simulink library "HY_General_Library"  (R2018b)
settings: Solver=ode45  StartTime=0.0  StopTime=10.0  RelTol=1e-3  EnableMultiTasking=on
undefined symbols (not defined in the file or in its folder): dT, Slope1, Slope2
libraries: simulink x63, $bdroot x4
(part 4 of 5)

== system HY_General_Library/PID_Blocks/IncrementalPID ==
  Err : Inport
  Kp : Inport  Port=2
  Ki : Inport  Port=3
  Kd : Inport  Port=4
  OutMax : Inport  Port=5
  OutMin : Inport  Port=6
  R : Inport  Port=7
  RV : Inport  Port=8
  Add : Sum  Inputs=+++
  Add1 : Sum  Inputs=+-
  Add2 : Sum
  Add3 : Sum  Inputs=+-
  Add4 : Sum  Inputs=+-
  Add5 : Sum
  Data Type Conversion : DataTypeConversion  OutDataTypeStr=single
  MinMax : MinMax  Inputs=2
  MinMax1 : MinMax  Function=max  Inputs=2
  Product : Product
  Product1 : Product
  Product2 : Product
  Switch : Switch  Criteria=u2 ~= 0
      settings: AttributesFormatString=%<Criteria>
  Unit Delay : UnitDelay  SampleTime=-1
      settings: AttributesFormatString=Init: %<X0>
  Unit Delay1 : UnitDelay  SampleTime=-1
      settings: AttributesFormatString=Init=%<X0>
  Unit Delay2 : UnitDelay  SampleTime=-1
      settings: AttributesFormatString=Init=%<X0>
  PIDOut : Outport
  POut : Outport  Port=2
  IOut : Outport  Port=3
  DOut : Outport  Port=4
  wires:
  Add2/1 -> Add1/1
  Kd/1 -> Product2/1
  Data Type Conversion/1 -> Unit Delay1/1, Add2/1, Product1/2, Add3/1
  Kp/1 -> Product/1
  Add4/1 -> Product2/2
  Ki/1 -> Product1/1
  Unit Delay1/1 -> Unit Delay2/1, Add1/2, Add4/2, Add3/2
  Add3/1 -> Product/2
  Product1/1 -> Add/2, IOut/1
  Product/1 -> Add/1, POut/1
  Product2/1 -> Add/3, DOut/1
  Err/1 -> Data Type Conversion/1
  OutMax/1 -> MinMax/1
  MinMax/1 -> MinMax1/1
  OutMin/1 -> MinMax1/2
  Unit Delay/1 -> Add5/2
  MinMax1/1 -> PIDOut/1, Unit Delay/1
  Add/1 -> Add5/1
  Add5/1 -> Switch/3
  Unit Delay2/1 -> Add2/2
  Add1/1 -> Add4/1
  Switch/1 -> MinMax/2
  R/1 -> Switch/2
  RV/1 -> Switch/1

== system HY_General_Library/PID_Blocks/PositionPID ==
  Err : Inport
  CtrlPropVal : Inport  Port=2
  CtrlIntgVal : Inport  Port=3
  CtrlDerivVal : Inport  Port=4
  UpperSatLimd : Inport  Port=5
  FfEnaFlag : Inport  Port=6
  FfVal : Inport  Port=7
  ThdMax : Inport  Port=8
  ThdMin : Inport  Port=9
  Reset : Inport  Port=10
  ResetVal : Inport  Port=11
  LowerSatLimd : Inport  Port=12
  Add : Sum  Inputs=+++
  Add3 : Sum  Inputs=+-
  Add4 : Sum
  MinMax : MinMax  Inputs=2
  MinMax1 : MinMax  Function=max  Inputs=2
  Product : Product
  Product2 : Product
  Subsystem1 : Subsystem
  Switch : Switch  Criteria=u2 ~= 0
  Unit Delay2 : UnitDelay  SampleTime=-1
  Output : Outport
  wires:
  Err/1 -> [Err], Product/1
  CtrlDerivVal/1 -> Product2/2
  [Err] -> Unit Delay2/1, Add3/1
  CtrlIntgVal/1 -> Subsystem1/5(CtrlIntgVal)
  ThdMax/1 -> MinMax/1
  Subsystem1/1(Out) -> Add/2
  Product/1 -> Add/1
  MinMax/1 -> MinMax1/1
  CtrlPropVal/1 -> Product/2
  FfVal/1 -> Add4/1
  Add/1 -> Switch/3, Add4/2
  Unit Delay2/1 -> Add3/2
  MinMax1/1 -> Output/1
  Add3/1 -> Product2/1
  Product2/1 -> Add/3
  ThdMin/1 -> MinMax1/2
  Reset/1 -> Subsystem1/1(Reset)
  [PreSat] -> Subsystem1/2(PreSat)
  UpperSatLimd/1 -> Subsystem1/3(UpperSatLimd)
  [Err] -> Subsystem1/4(Err)
  Switch/1 -> [PreSat], MinMax/2
  Add4/1 -> Switch/1
  FfEnaFlag/1 -> Switch/2
  ResetVal/1 -> Subsystem1/6(ResetVal)
  LowerSatLimd/1 -> Subsystem1/7(LowerSatLimd)

== system HY_General_Library/Time&Counter_Blocks/BounceTimer ==
  TmrEna : Inport
  Inc : Inport  Port=2
  MaxTime : Inport  Port=3
  Add : Sum
  Constant : Constant  Value=uint16(0)
  Multiport Switch1 : MultiPortSwitch  DataPortOrder=Zero-based contiguous  Inputs=2  zeroidx=on  OutDataTypeStr=double
  Relational Operator : RelationalOperator  OutDataTypeStr=boolean  RndMeth=Nearest
  Unit Delay1 : UnitDelay  SampleTime=-1
  TrigOut : Outport
  Timer : Outport  Port=2
  wires:
  Constant/1 -> Multiport Switch1/2
  TmrEna/1 -> Multiport Switch1/1
  MaxTime/1 -> Relational Operator/2
  Inc/1 -> Add/1
  Multiport Switch1/1 -> Add/2, Timer/1, Relational Operator/1
  Add/1 -> Unit Delay1/1
  Unit Delay1/1 -> Multiport Switch1/3
  Relational Operator/1 -> TrigOut/1

== system HY_General_Library/Time&Counter_Blocks/COUNTER ==
  E : Inport  OutDataTypeStr=boolean
  Constant1 : Constant  OutDataTypeStr=uint32
  Constant3 : Constant  Value=0  OutDataTypeStr=uint32
  Constant4 : Constant  Value=limit_value  OutDataTypeStr=uint32
  Min : MinMax  Inputs=2  SaturateOnIntegerOverflow=on
  Sum1 : Sum  SaturateOnIntegerOverflow=on
  Switch1 : Switch  Criteria=u2 ~= 0  Threshold=0.5  SaturateOnIntegerOverflow=on  InputSameDT=on
      settings: AttributesFormatString=%<Criteria>
  Unit Delay : UnitDelay  SampleTime=-1
      settings: AttributesFormatString=Init: %<X0>
  y : Outport
  wires:
  E/1 -> Switch1/2
  Sum1/1 -> Min/2
  Unit Delay/1 -> Sum1/1
  Constant3/1 -> Switch1/3
  Switch1/1 -> y/1, Unit Delay/1
  Min/1 -> Switch1/1
  Constant4/1 -> Min/1
  Constant1/1 -> Sum1/2

== system HY_General_Library/Time&Counter_Blocks/COUNTER_H ==
  E : Inport  OutDataTypeStr=boolean
  R : Inport  Port=2  OutDataTypeStr=boolean
  Constant1 : Constant  OutDataTypeStr=uint32
  Constant2 : Constant  Value=0  OutDataTypeStr=uint32
  Constant3 : Constant  Value=0  OutDataTypeStr=uint32
  Constant4 : Constant  Value=limit_value  OutDataTypeStr=uint32
  MinMax : MinMax  Inputs=2  SaturateOnIntegerOverflow=on
  Sum1 : Sum  SaturateOnIntegerOverflow=on
  Switch : Switch  Criteria=u2 ~= 0  Threshold=0.5
  Switch1 : Switch  Criteria=u2 ~= 0  Threshold=0.5  SaturateOnIntegerOverflow=on  InputSameDT=on
      settings: AttributesFormatString=%<Criteria>
  Unit Delay : UnitDelay  SampleTime=-1
      settings: AttributesFormatString=Init: %<X0>
  y : Outport
  wires:
  Unit Delay/1 -> Sum1/2
  Switch/1 -> Sum1/1
  Constant3/1 -> Switch1/1
  MinMax/1 -> Switch1/3
  Constant4/1 -> MinMax/1
  Switch1/1 -> Unit Delay/1, y/1
  Constant2/1 -> Switch/3
  Sum1/1 -> MinMax/2
  Constant1/1 -> Switch/1
  E/1 -> Switch/2
  R/1 -> Switch1/2

== system HY_General_Library/Time&Counter_Blocks/STOPWATCH_RE ==
  E : Inport  OutDataTypeStr=boolean
  R : Inport  Port=2  OutDataTypeStr=boolean
  dT : Inport  Port=3
  Constant1 : Constant  Value=0.0  OutDataTypeStr=Inherit: Inherit via back propagation
  Sum1 : Sum  SaturateOnIntegerOverflow=on
  Switch : Switch  Criteria=u2 ~= 0  SaturateOnIntegerOverflow=on  InputSameDT=on
  Switch1 : Switch  Criteria=u2 ~= 0  SaturateOnIntegerOverflow=on  InputSameDT=on
  Unit Delay1 : UnitDelay  SampleTime=-1
      settings: AttributesFormatString=<initial=%<x0>>
  t : Outport
  wires:
  Sum1/1 -> Switch1/1
  Unit Delay1/1 -> Switch1/3, Sum1/2
  R/1 -> Switch/2
  Constant1/1 -> Switch/1
  E/1 -> Switch1/2
  Switch1/1 -> Switch/3
  Switch/1 -> t/1, Unit Delay1/1
  dT/1 -> Sum1/1

== system HY_General_Library/Time&Counter_Blocks/TIMER ==
  T : Inport
  S : Inport  Port=2  OutDataTypeStr=boolean
  dT : Inport  Port=3
  Constant3 : Constant  Value=0.0001  OutDataTypeStr=Inherit: Inherit via back propagation
  Constant5 : Constant  Value=0  OutDataTypeStr=Inherit: Inherit via back propagation
  Logical Operator1 : Logic  Operator=NOT  Inputs=1  OutDataTypeStr=boolean
  Logical Operator2 : Logic  OutDataTypeStr=boolean
  Logical Operator4 : Logic  Operator=NOT  Inputs=1  OutDataTypeStr=boolean
  Logical Operator5 : Logic  OutDataTypeStr=boolean
  Logical Operator7 : Logic  Operator=OR  OutDataTypeStr=boolean
  MinMax : MinMax  Inputs=2  SaturateOnIntegerOverflow=on  InputSameDT=on
  Relational Operator : RelationalOperator  Operator=<=  OutDataTypeStr=boolean  RndMeth=Nearest  InputSameDT=on
  Sum : Sum  SaturateOnIntegerOverflow=on
  Sum1 : Sum  SaturateOnIntegerOverflow=on
  Switch2 : Switch  Criteria=u2 ~= 0  Threshold=0.5  SaturateOnIntegerOverflow=on  InputSameDT=on
  Switch3 : Switch  Criteria=u2 ~= 0  Threshold=0.5  SaturateOnIntegerOverflow=on  InputSameDT=on
  Unit Delay : UnitDelay  SampleTime=-1
      settings: AttributesFormatString=<initial=%<x0>>
  Unit Delay1 : UnitDelay  SampleTime=-1
      settings: AttributesFormatString=<initial=%<x0>>
  Unit Delay2 : UnitDelay  SampleTime=-1
      settings: AttributesFormatString=<initial=%<x0>>
  y : Outport
  t : Outport  Port=2
  wires:
  Logical Operator1/1 -> Logical Operator7/2
  Logical Operator4/1 -> Logical Operator5/2
  T/1 -> Switch3/1
  Sum/1 -> Switch2/3
  Unit Delay1/1 -> Logical Operator4/1
  Constant5/1 -> Switch2/1
  Sum1/1 -> Relational Operator/2
  Logical Operator2/1 -> y/1
  Constant3/1 -> Sum1/1
  Relational Operator/1 -> Logical Operator2/2
  S/1 -> Logical Operator2/1, Unit Delay1/1, Logical Operator5/1, Logical Operator1/1
  Switch3/1 -> Relational Operator/1, MinMax/1, Unit Delay2/1  "sampled_target_time"
  Unit Delay2/1 -> Switch3/3
  Switch2/1 -> MinMax/2
  Logical Operator7/1 -> Switch2/2
  dT/1 -> Sum/1
  Logical Operator5/1 -> Switch3/2, Logical Operator7/1  "edge"
  Unit Delay/1 -> Sum/2  "timer_value_old"
  MinMax/1 -> t/1, Unit Delay/1, Sum1/2

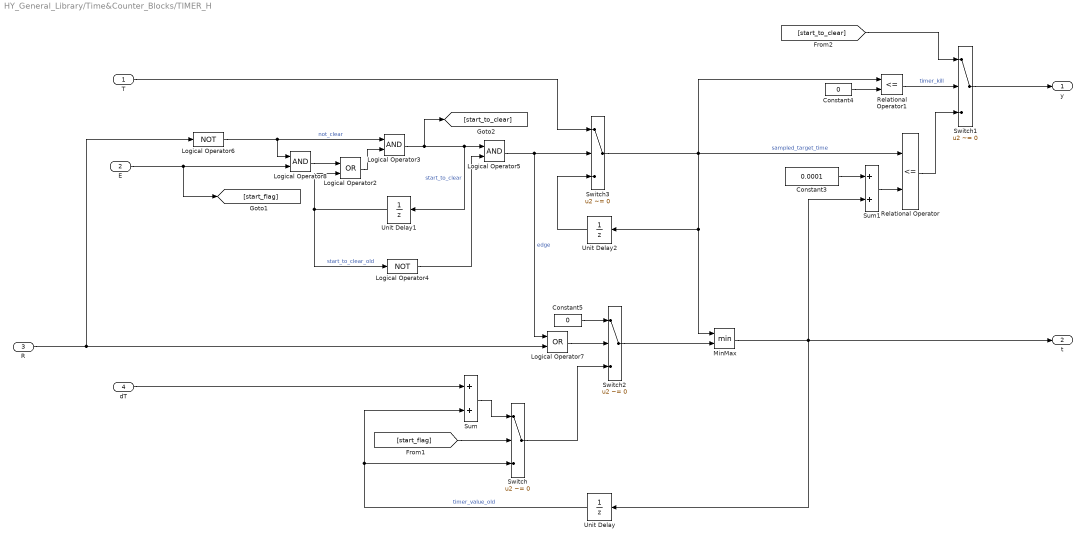
== system HY_General_Library/Time&Counter_Blocks/TIMER_H ==
  T : Inport
  E : Inport  Port=2  OutDataTypeStr=boolean
  R : Inport  Port=3  OutDataTypeStr=boolean
  dT : Inport  Port=4
  Constant3 : Constant  Value=0.0001  OutDataTypeStr=Inherit: Inherit via back propagation
  Constant4 : Constant  Value=0  OutDataTypeStr=Inherit: Inherit via back propagation
  Constant5 : Constant  Value=0  OutDataTypeStr=Inherit: Inherit via back propagation
  Logical Operator2 : Logic  Operator=OR  OutDataTypeStr=boolean
  Logical Operator3 : Logic  OutDataTypeStr=boolean
  Logical Operator4 : Logic  Operator=NOT  Inputs=1  OutDataTypeStr=boolean
  Logical Operator5 : Logic  OutDataTypeStr=boolean
  Logical Operator6 : Logic  Operator=NOT  Inputs=1  OutDataTypeStr=boolean
  Logical Operator7 : Logic  Operator=OR  OutDataTypeStr=boolean
  Logical Operator8 : Logic  OutDataTypeStr=boolean
  MinMax : MinMax  Inputs=2  SaturateOnIntegerOverflow=on  InputSameDT=on
  Relational Operator : RelationalOperator  Operator=<=  OutDataTypeStr=boolean  RndMeth=Nearest  InputSameDT=on
  Relational Operator1 : RelationalOperator  Operator=<=  OutDataTypeStr=boolean  RndMeth=Nearest  InputSameDT=on
  Sum : Sum  SaturateOnIntegerOverflow=on
  Sum1 : Sum  SaturateOnIntegerOverflow=on
  Switch{,1..3} (4 alike) : Switch  Criteria=u2 ~= 0  Threshold=0.5  SaturateOnIntegerOverflow=on  InputSameDT=on
  Unit Delay : UnitDelay  SampleTime=-1
      settings: AttributesFormatString=<initial=%<x0>>
  Unit Delay1 : UnitDelay  SampleTime=-1
      settings: AttributesFormatString=<initial=%<x0>>
  Unit Delay2 : UnitDelay  SampleTime=-1
      settings: AttributesFormatString=<initial=%<x0>>
  y : Outport
  t : Outport  Port=2
  wires:
  [start_to_clear] -> Switch1/1
  E/1 -> Logical Operator8/2, [start_flag]
  MinMax/1 -> Sum1/2, Unit Delay/1, t/1
  Unit Delay/1 -> Switch/3, Sum/2  "timer_value_old"
  R/1 -> Logical Operator6/1, Logical Operator7/2
  Logical Operator8/1 -> Logical Operator2/1
  [start_flag] -> Switch/2
  Logical Operator6/1 -> Logical Operator8/1, Logical Operator3/1  "not_clear"
  T/1 -> Switch3/1
  Logical Operator5/1 -> Logical Operator7/1, Switch3/2  "edge"
  Logical Operator4/1 -> Logical Operator5/2
  Unit Delay1/1 -> Logical Operator4/1, Logical Operator2/2  "start_to_clear_old"
  Logical Operator3/1 -> [start_to_clear], Logical Operator5/1, Unit Delay1/1  "start_to_clear"
  Logical Operator2/1 -> Logical Operator3/2
  dT/1 -> Sum/1
  Sum/1 -> Switch/1
  Switch/1 -> Switch2/3
  Logical Operator7/1 -> Switch2/2
  Switch2/1 -> MinMax/2
  Unit Delay2/1 -> Switch3/3
  Switch3/1 -> Relational Operator1/1, Unit Delay2/1, MinMax/1, Relational Operator/1  "sampled_target_time"
  Relational Operator/1 -> Switch1/3
  Constant3/1 -> Sum1/1
  Relational Operator1/1 -> Switch1/2  "timer_kill"
  Switch1/1 -> y/1
  Constant4/1 -> Relational Operator1/2
  Sum1/1 -> Relational Operator/2
  Constant5/1 -> Switch2/1

== system HY_General_Library/Time&Counter_Blocks/TIME_Y ==
  T : Inport
  S : Inport  Port=2  OutDataTypeStr=boolean
  dT : Inport  Port=3
  Constant3 : Constant  Value=0.0001  OutDataTypeStr=Inherit: Inherit via back propagation
  Constant5 : Constant  Value=0  OutDataTypeStr=Inherit: Inherit via back propagation
  Logical Operator1 : Logic  Operator=NOT  Inputs=1  OutDataTypeStr=boolean
  Logical Operator2 : Logic  OutDataTypeStr=boolean
  Logical Operator4 : Logic  Operator=NOT  Inputs=1  OutDataTypeStr=boolean
  Logical Operator5 : Logic  OutDataTypeStr=boolean
  Logical Operator7 : Logic  Operator=OR  OutDataTypeStr=boolean
  MinMax : MinMax  Inputs=2  SaturateOnIntegerOverflow=on  InputSameDT=on
  Relational Operator : RelationalOperator  Operator=<=  OutDataTypeStr=boolean  RndMeth=Nearest  InputSameDT=on
  Sum : Sum  SaturateOnIntegerOverflow=on
  Sum1 : Sum  SaturateOnIntegerOverflow=on
  Switch2 : Switch  Criteria=u2 ~= 0  Threshold=0.5  SaturateOnIntegerOverflow=on  InputSameDT=on
  Switch3 : Switch  Criteria=u2 ~= 0  Threshold=0.5  SaturateOnIntegerOverflow=on  InputSameDT=on
  Unit Delay : UnitDelay  SampleTime=-1
      settings: AttributesFormatString=<initial=%<x0>>
  Unit Delay1 : UnitDelay  SampleTime=-1
      settings: AttributesFormatString=<initial=%<x0>>
  Unit Delay2 : UnitDelay  SampleTime=-1
      settings: AttributesFormatString=<initial=%<x0>>
  y : Outport
  wires:
  MinMax/1 -> Sum1/2, Unit Delay/1
  Unit Delay/1 -> Sum/2  "timer_value_old"
  Logical Operator5/1 -> Logical Operator7/1, Switch3/2  "edge"
  dT/1 -> Sum/1
  Logical Operator7/1 -> Switch2/2
  Switch2/1 -> MinMax/2
  Unit Delay2/1 -> Switch3/3
  Switch3/1 -> Unit Delay2/1, MinMax/1, Relational Operator/1  "sampled_target_time"
  S/1 -> Logical Operator1/1, Logical Operator5/1, Unit Delay1/1, Logical Operator2/1
  Relational Operator/1 -> Logical Operator2/2
  Constant3/1 -> Sum1/1
  Logical Operator2/1 -> y/1
  Sum1/1 -> Relational Operator/2
  Constant5/1 -> Switch2/1
  Unit Delay1/1 -> Logical Operator4/1
  Sum/1 -> Switch2/3
  T/1 -> Switch3/1
  Logical Operator4/1 -> Logical Operator5/2
  Logical Operator1/1 -> Logical Operator7/2

== system HY_General_Library/Time&Counter_Blocks/TurnOffDelay ==
  u : Inport
  T : Inport  Port=2
  dT : Inport  Port=3
  Dif : Sum  Inputs=+-  SaturateOnIntegerOverflow=on
  Logical Operator1 : Logic  Operator=OR  OutDataTypeStr=boolean
  Relational Operator : RelationalOperator  Operator=>  OutDataTypeStr=boolean  RndMeth=Nearest  InputSameDT=on
  Switch : Switch  Criteria=u2 ~= 0  SaturateOnIntegerOverflow=on  InputSameDT=on
  Switch1 : Switch  Criteria=u2 ~= 0  SaturateOnIntegerOverflow=on  InputSameDT=on
  Unit Delay1 : UnitDelay  SampleTime=-1
      settings: AttributesFormatString=<initial=%<x0>>
  Zero_C : Constant  Value=0.0  OutDataTypeStr=Inherit: Inherit via back propagation
  y : Outport  InitialOutput=0
  wires:
  u/1 -> Switch/2, Logical Operator1/2
  Unit Delay1/1 -> Dif/1, Relational Operator/1, Switch1/3
  T/1 -> Switch/1
  Relational Operator/1 -> Logical Operator1/1, Switch1/2
  Logical Operator1/1 -> y/1
  Switch/1 -> Unit Delay1/1
  Zero_C/1 -> Relational Operator/2
  Switch1/1 -> Switch/3
  dT/1 -> Dif/2
  Dif/1 -> Switch1/1

== system HY_General_Library/Time&Counter_Blocks/TurnOffDelayCnt ==
  u : Inport
  Cnt : Inport  Port=2
  Constant1 : Constant  Value=0  OutDataTypeStr=Inherit: Inherit via back propagation
  Constant2 : Constant  OutDataTypeStr=Inherit: Inherit via back propagation
  Constant3 : Constant  Value=0  OutDataTypeStr=Inherit: Inherit via back propagation
  Data Type Duplicate : DataTypeDuplicate  NumInputPorts=4
  Logical Operator : Logic  OutDataTypeStr=boolean
  Logical Operator1 : Logic  OutDataTypeStr=boolean
  Logical Operator2 : Logic  Operator=NOT  OutDataTypeStr=boolean
  RelationalOperator : RelationalOperator  RndMeth=Nearest  InputSameDT=on
  Sum : Sum  SaturateOnIntegerOverflow=on
  Switch1 : Switch  Criteria=u2 ~= 0  SaturateOnIntegerOverflow=on  InputSameDT=on
      settings: AttributesFormatString=%<Criteria>
  Switch4 : Switch  Criteria=u2 ~= 0  SaturateOnIntegerOverflow=on  InputSameDT=on
      settings: AttributesFormatString=%<Criteria>
  Unit Delay : UnitDelay  SampleTime=-1
      settings: AttributesFormatString=Init: %<X0>
  Unit Delay1 : UnitDelay  SampleTime=-1
      settings: AttributesFormatString=Init: %<X0>
  y : Outport
  wires:
  [u] -> Logical Operator/2
  Switch1/1 -> Sum/1
  Constant3/1 -> Switch1/3, Data Type Duplicate/2
  [u] -> Switch1/2
  Unit Delay/1 -> Switch1/1
  Switch4/1 -> Sum/2
  Constant2/1 -> Switch4/1, Data Type Duplicate/3
  Constant1/1 -> Switch4/3, Data Type Duplicate/4
  Logical Operator2/1 -> Logical Operator1/1
  Logical Operator1/1 -> Switch4/2
  Unit Delay1/1 -> Logical Operator2/1
  Cnt/1 -> RelationalOperator/2, Data Type Duplicate/1
  Sum/1 -> Unit Delay/1, RelationalOperator/1
  Logical Operator/1 -> y/1
  RelationalOperator/1 -> Logical Operator/1, Unit Delay1/1
  u/1 -> [u], Logical Operator1/2

== system HY_General_Library/Time&Counter_Blocks/TurnOffDelay_R ==
  u : Inport
  R : Inport  Port=2
  T : Inport  Port=3
  dT : Inport  Port=4
  Data Type Duplicate : DataTypeDuplicate  NumInputPorts=4
  Dif : Sum  Inputs=+-  SaturateOnIntegerOverflow=on
  Logical Operator1 : Logic  Operator=OR  OutDataTypeStr=boolean
  Logical Operator2 : Logic
  Logical Operator3 : Logic  Operator=NOT  Inputs=1  AllPortsSameDT=off  OutDataTypeStr=boolean
  Relational Operator : RelationalOperator  Operator=>  OutDataTypeStr=boolean  RndMeth=Nearest  InputSameDT=on
  Switch : Switch  Criteria=u2 ~= 0  SaturateOnIntegerOverflow=on  InputSameDT=on
      settings: AttributesFormatString=%<Criteria>
  Switch1 : Switch  Criteria=u2 ~= 0  SaturateOnIntegerOverflow=on  InputSameDT=on
      settings: AttributesFormatString=%<Criteria>
  Switch2 : Switch  Criteria=u2 ~= 0  SaturateOnIntegerOverflow=on  InputSameDT=on
      settings: AttributesFormatString=%<Criteria>
  Unit Delay1 : UnitDelay  SampleTime=-1
      settings: AttributesFormatString=Init: %<X0>
  Zero_C : Constant  Value=0  OutDataTypeStr=Inherit: Inherit via back propagation
  Zero_C1 : Constant  Value=0  OutDataTypeStr=single
      settings: AttributesFormatString=%<OutDataTypeStr>
  y : Outport  InitialOutput=0
  wires:
  Logical Operator2/1 -> Logical Operator1/2, Switch/2
  Switch2/1 -> Switch1/3, Relational Operator/1, Dif/1
  T/1 -> Switch/1, Data Type Duplicate/4
  Relational Operator/1 -> Logical Operator1/1, Switch1/2
  Logical Operator1/1 -> y/1
  Switch/1 -> Unit Delay1/1
  Zero_C/1 -> Data Type Duplicate/1, Relational Operator/2
  Switch1/1 -> Switch/3
  dT/1 -> Data Type Duplicate/2, Dif/2
  Dif/1 -> Switch1/1
  u/1 -> Logical Operator2/2
  Logical Operator3/1 -> Logical Operator2/1
  R/1 -> Logical Operator3/1, Switch2/2
  Unit Delay1/1 -> Switch2/3
  Zero_C1/1 -> Switch2/1, Data Type Duplicate/3

== system HY_General_Library/Time&Counter_Blocks/TurnOnDelay ==
  u : Inport
  T : Inport  Port=2
  dT : Inport  Port=3
  Constant1 : Constant  Value=0.0  OutDataTypeStr=Inherit: Inherit via back propagation
  Logical Operator : Logic  OutDataTypeStr=boolean
  Logical Operator2 : Logic  Operator=NOT  Inputs=1  AllPortsSameDT=off  OutDataTypeStr=boolean
  Logical Operator3 : Logic  Operator=NOT  Inputs=1  AllPortsSameDT=off  OutDataTypeStr=boolean
  Logical Operator4 : Logic  Operator=NOT  Inputs=1  AllPortsSameDT=off  OutDataTypeStr=boolean
  Relational Operator2 : RelationalOperator  Operator=>  OutDataTypeStr=boolean  RndMeth=Nearest  InputSameDT=on
  Sum : Sum  Inputs=+-  SaturateOnIntegerOverflow=on
  Switch : Switch  Criteria=u2 ~= 0  SaturateOnIntegerOverflow=on  InputSameDT=on
      settings: AttributesFormatString=%<Criteria>
  Switch4 : Switch  Criteria=u2 ~= 0  SaturateOnIntegerOverflow=on  InputSameDT=on
      settings: AttributesFormatString=%<Criteria>
  Unit Delay : UnitDelay  SampleTime=-1
      settings: AttributesFormatString=Init: %<X0>
  y : Outport
  wires:
  Logical Operator2/1 -> Switch/2
  Switch4/1 -> Unit Delay/1
  Sum/1 -> Switch/3
  dT/1 -> Sum/2
  Constant1/1 -> Relational Operator2/2
  Relational Operator2/1 -> Logical Operator2/1, Logical Operator3/1
  u/1 -> Logical Operator4/1, Logical Operator/2
  Logical Operator/1 -> y/1
  Switch/1 -> Switch4/3
  Logical Operator3/1 -> Logical Operator/1
  Logical Operator4/1 -> Switch4/2
  T/1 -> Switch4/1
  Unit Delay/1 -> Relational Operator2/1, Switch/1, Sum/1

== system HY_General_Library/Time&Counter_Blocks/TurnOnDelayCnt ==
  u : Inport
  Cnt : Inport  Port=2
  Constant1 : Constant  Value=0  OutDataTypeStr=Inherit: Inherit via back propagation
  Constant2 : Constant  OutDataTypeStr=Inherit: Inherit via back propagation
  Constant3 : Constant  Value=0  OutDataTypeStr=Inherit: Inherit via back propagation
  Data Type Duplicate : DataTypeDuplicate  NumInputPorts=4
  Logical Operator : Logic  OutDataTypeStr=boolean
  Logical Operator1 : Logic  OutDataTypeStr=boolean
  Logical Operator2 : Logic  Operator=NOT  OutDataTypeStr=boolean
  RelationalOperator : RelationalOperator  RndMeth=Nearest  InputSameDT=on
  Sum : Sum  SaturateOnIntegerOverflow=on
  Switch1 : Switch  Criteria=u2 ~= 0  SaturateOnIntegerOverflow=on  InputSameDT=on
      settings: AttributesFormatString=%<Criteria>
  Switch4 : Switch  Criteria=u2 ~= 0  SaturateOnIntegerOverflow=on  InputSameDT=on
      settings: AttributesFormatString=%<Criteria>
  Unit Delay : UnitDelay  SampleTime=-1
      settings: AttributesFormatString=Init: %<X0>
  Unit Delay1 : UnitDelay  SampleTime=-1
      settings: AttributesFormatString=Init: %<X0>
  y : Outport
  wires:
  u/1 -> Logical Operator1/2, [u]
  RelationalOperator/1 -> Unit Delay1/1, Logical Operator/1
  Logical Operator/1 -> y/1
  Sum/1 -> RelationalOperator/1, Unit Delay/1
  Cnt/1 -> Data Type Duplicate/1, RelationalOperator/2
  Unit Delay1/1 -> Logical Operator2/1
  Logical Operator1/1 -> Switch4/2
  Logical Operator2/1 -> Logical Operator1/1
  Constant1/1 -> Data Type Duplicate/4, Switch4/3
  Constant2/1 -> Data Type Duplicate/3, Switch4/1
  Switch4/1 -> Sum/2
  Unit Delay/1 -> Switch1/1
  [u] -> Switch1/2
  Constant3/1 -> Data Type Duplicate/2, Switch1/3
  Switch1/1 -> Sum/1
  [u] -> Logical Operator/2

== system HY_General_Library/Time&Counter_Blocks/TurnOnDelay_IV ==
  u : Inport
  T : Inport  Port=2
  dT : Inport  Port=3
  IV : Inport  Port=4
  Constant : Constant  Value=boolean(0)  OutDataTypeStr=boolean
  Constant1 : Constant  Value=0.0  OutDataTypeStr=Inherit: Inherit via back propagation
  Logical Operator : Logic  OutDataTypeStr=boolean
  Logical Operator2 : Logic  Operator=NOT  Inputs=1  AllPortsSameDT=off  OutDataTypeStr=boolean
  Logical Operator3 : Logic  Operator=NOT  Inputs=1  AllPortsSameDT=off  OutDataTypeStr=boolean
  Logical Operator4 : Logic  Operator=NOT  Inputs=1  AllPortsSameDT=off  OutDataTypeStr=boolean
  Relational Operator2 : RelationalOperator  Operator=>  RndMeth=Nearest  InputSameDT=on
  Sum : Sum  Inputs=+-  SaturateOnIntegerOverflow=on
  Switch : Switch  Criteria=u2 ~= 0  SaturateOnIntegerOverflow=on  InputSameDT=on
  Switch1 : Switch  Criteria=u2 ~= 0  SaturateOnIntegerOverflow=on  InputSameDT=on
  Switch4 : Switch  Criteria=u2 ~= 0  SaturateOnIntegerOverflow=on  InputSameDT=on
  Unit Delay : UnitDelay  SampleTime=-1
      settings: AttributesFormatString=<initial=%<x0>>
  Unit Delay1 : UnitDelay  InitialCondition=1  SampleTime=-1
  y : Outport
  wires:
  Unit Delay/1 -> Sum/1, Switch/1, Relational Operator2/1
  T/1 -> Switch4/1
  Logical Operator4/1 -> Switch4/2
  Logical Operator3/1 -> Logical Operator/1
  Switch/1 -> Switch4/3
  Switch1/1 -> y/1
  u/1 -> Logical Operator/2, Logical Operator4/1
  Relational Operator2/1 -> Logical Operator3/1, Logical Operator2/1
  Constant1/1 -> Relational Operator2/2
  dT/1 -> Sum/2
  Sum/1 -> Switch/3
  Switch4/1 -> Unit Delay/1
  Logical Operator2/1 -> Switch/2
  Logical Operator/1 -> Switch1/3
  Unit Delay1/1 -> Switch1/2
  Constant/1 -> Unit Delay1/1
  IV/1 -> Switch1/1

== system HY_General_Library/Trigger_Blocks/EVENT ==
  Constant1 : Constant  Value=EventTime  OutDataTypeStr=Inherit: Inherit via back propagation
  Constant2 : Constant  Value=0  OutDataTypeStr=Inherit: Inherit via back propagation
  Constant3 : Constant  Value=0.0001  OutDataTypeStr=Inherit: Inherit via back propagation
  Constant4 : Constant  Value=SampleTime  OutDataTypeStr=Inherit: Inherit via back propagation
  Relational Operator1 : RelationalOperator  Operator=<  OutDataTypeStr=boolean  RndMeth=Nearest  InputSameDT=on
  Sum1 : Sum  SaturateOnIntegerOverflow=on
  Sum2 : Sum  Inputs=++-  SaturateOnIntegerOverflow=on
  Switch1 : Switch  Criteria=u2 ~= 0  Threshold=0.5  OutDataTypeStr=Inherit: Inherit via back propagation  SaturateOnIntegerOverflow=on
  Unit Delay1 : UnitDelay  SampleTime=-1
      settings: AttributesFormatString=Init: %<X0>
  event : Outport
  wires:
  Constant3/1 -> Sum2/2
  Relational Operator1/1 -> Switch1/2, event/1
  Sum1/1 -> Relational Operator1/2, Switch1/3
  Constant4/1 -> Sum2/3, Sum1/1
  Sum2/1 -> Relational Operator1/1
  Unit Delay1/1 -> Sum1/2
  Constant1/1 -> Sum2/1
  Constant2/1 -> Switch1/1
  Switch1/1 -> Unit Delay1/1

== system HY_General_Library/Trigger_Blocks/PWM ==
  ONT : Inport
  OFFT : Inport  Port=2
  En : Inport  Port=3
  ST : Inport  Port=4
  Constant1 : Constant  Value=0  OutDataTypeStr=Inherit: Inherit via back propagation
  Constant2 : Constant  Value=0  OutDataTypeStr=Inherit: Inherit via back propagation
  Constant3 : Constant  Value=0.0001  OutDataTypeStr=Inherit: Inherit via back propagation
  Logical Operator : Logic  Operator=OR  AllPortsSameDT=off  OutDataTypeStr=boolean
  Logical Operator1 : Logic  Operator=NOT  Inputs=1  AllPortsSameDT=off  OutDataTypeStr=boolean
  Relational Operator1 : RelationalOperator  Operator=>  OutDataTypeStr=boolean  RndMeth=Nearest  InputSameDT=on
  Relational Operator2 : RelationalOperator  Operator=<  OutDataTypeStr=boolean  RndMeth=Nearest  InputSameDT=on
  Sum1 : Sum  SaturateOnIntegerOverflow=on
  Sum3 : Sum  SaturateOnIntegerOverflow=on
  Sum4 : Sum  SaturateOnIntegerOverflow=on
  Sum5 : Sum  Inputs=+-  SaturateOnIntegerOverflow=on
  Switch1 : Switch  Criteria=u2 ~= 0  Threshold=0.5  OutDataTypeStr=Inherit: Inherit via back propagation  SaturateOnIntegerOverflow=on
  Switch2 : Switch  Criteria=u2 ~= 0  Threshold=0.5  OutDataTypeStr=Inherit: Inherit via back propagation  SaturateOnIntegerOverflow=on
  Unit Delay1 : UnitDelay  SampleTime=-1
      settings: AttributesFormatString=<initial=%<x0>>
  PWM : Outport
  wires:
  Switch1/1 -> Unit Delay1/1
  Unit Delay1/1 -> Sum1/2
  Sum5/1 -> Sum4/2
  Sum1/1 -> Switch1/3, Relational Operator2/2, Relational Operator1/2  "timer"
  Relational Operator1/1 -> PWM/1  "PWM"
  Constant3/1 -> Sum3/2
  Constant2/1 -> Switch2/3
  ST/1 -> Sum5/2, Sum1/1
  ONT/1 -> Switch2/1
  En/1 -> Logical Operator1/1, Switch2/2
  Switch2/1 -> Sum3/1
  OFFT/1 -> Sum4/1
  Sum4/1 -> Relational Operator2/1  "OffTarget"
  Relational Operator2/1 -> Logical Operator/1
  Constant1/1 -> Switch1/1
  Logical Operator/1 -> Switch1/2
  Logical Operator1/1 -> Logical Operator/2
  Sum3/1 -> Relational Operator1/1, Sum5/1  "OnTarget"

== system HY_General_Library/Algebric_Blocks/DIVIDE/Subsystem ==
  In1 : Inport
  In2 : Inport  Port=2
  Relational Operator2 : RelationalOperator  Operator=<=  OutDataTypeStr=boolean  RndMeth=Nearest  InputSameDT=on
  Switch1 : Switch  Criteria=u2 ~= 0
  MinOut : Outport
  wires:
  In2/1 -> Switch1/3, Relational Operator2/2
  Switch1/1 -> MinOut/1
  In1/1 -> Switch1/1, Relational Operator2/1
  Relational Operator2/1 -> Switch1/2

== system HY_General_Library/Algebric_Blocks/DIVIDE/Subsystem1 ==
  In1 : Inport
  In2 : Inport  Port=2
  Relational Operator2 : RelationalOperator  OutDataTypeStr=boolean  RndMeth=Nearest  InputSameDT=on
  Switch1 : Switch  Criteria=u2 ~= 0  InputSameDT=on
  MaxOut : Outport
  wires:
  Relational Operator2/1 -> Switch1/2
  In1/1 -> Switch1/1, Relational Operator2/1
  Switch1/1 -> MaxOut/1
  In2/1 -> Switch1/3, Relational Operator2/2

== system HY_General_Library/Debounce_Blocks/DebounceJump/TIMER ==
  T : Inport
  S : Inport  Port=2  OutDataTypeStr=boolean
  dT : Inport  Port=3
  Constant3 : Constant  Value=0.0001  OutDataTypeStr=Inherit: Inherit via back propagation
  Constant5 : Constant  Value=0  OutDataTypeStr=Inherit: Inherit via back propagation
  Logical Operator1 : Logic  Operator=NOT  Inputs=1  OutDataTypeStr=boolean
  Logical Operator2 : Logic  OutDataTypeStr=boolean
  Logical Operator4 : Logic  Operator=NOT  Inputs=1  OutDataTypeStr=boolean
  Logical Operator5 : Logic  OutDataTypeStr=boolean
  Logical Operator7 : Logic  Operator=OR  OutDataTypeStr=boolean
  MinMax : MinMax  Inputs=2  SaturateOnIntegerOverflow=on  InputSameDT=on
  Relational Operator : RelationalOperator  Operator=<=  OutDataTypeStr=boolean  RndMeth=Nearest  InputSameDT=on
  Sum : Sum  SaturateOnIntegerOverflow=on
  Sum1 : Sum  SaturateOnIntegerOverflow=on
  Switch2 : Switch  Criteria=u2 ~= 0  Threshold=0.5  SaturateOnIntegerOverflow=on  InputSameDT=on
  Switch3 : Switch  Criteria=u2 ~= 0  Threshold=0.5  SaturateOnIntegerOverflow=on  InputSameDT=on
  Unit Delay : UnitDelay  SampleTime=-1
      settings: AttributesFormatString=<initial=%<x0>>
  Unit Delay1 : UnitDelay  SampleTime=-1
      settings: AttributesFormatString=<initial=%<x0>>
  Unit Delay2 : UnitDelay  SampleTime=-1
      settings: AttributesFormatString=<initial=%<x0>>
  y : Outport
  wires:
  MinMax/1 -> Sum1/2, Unit Delay/1
  Unit Delay/1 -> Sum/2  "timer_value_old"
  Logical Operator5/1 -> Logical Operator7/1, Switch3/2  "edge"
  dT/1 -> Sum/1
  Logical Operator7/1 -> Switch2/2
  Switch2/1 -> MinMax/2
  Unit Delay2/1 -> Switch3/3
  Switch3/1 -> Unit Delay2/1, MinMax/1, Relational Operator/1  "sampled_target_time"
  S/1 -> Logical Operator1/1, Logical Operator5/1, Unit Delay1/1, Logical Operator2/1
  Relational Operator/1 -> Logical Operator2/2
  Constant3/1 -> Sum1/1
  Logical Operator2/1 -> y/1
  Sum1/1 -> Relational Operator/2
  Constant5/1 -> Switch2/1
  Unit Delay1/1 -> Logical Operator4/1
  Sum/1 -> Switch2/3
  T/1 -> Switch3/1
  Logical Operator4/1 -> Logical Operator5/2
  Logical Operator1/1 -> Logical Operator7/2

== system HY_General_Library/Debounce_Blocks/Debounce_Cnt/RS_FF_IV_Pos ==
  S : Inport  OutDataTypeStr=boolean
  R : Inport  Port=2  OutDataTypeStr=boolean
  IV : Inport  Port=3  OutDataTypeStr=boolean
  AND : Logic  OutDataTypeStr=boolean
  Constant : Constant  Value=0  OutDataTypeStr=boolean
      settings: AttributesFormatString=%<OutDataTypeStr>
  NOT : Logic  Operator=NOT  Inputs=1  OutDataTypeStr=boolean
  OR : Logic  Operator=OR  OutDataTypeStr=boolean
  Switch : Switch  Criteria=u2 ~= 0  InputSameDT=on
      settings: AttributesFormatString=|
      | %<Criteria>
      | Threshold=%<Threshold>
  Unit Delay : UnitDelay  SampleTime=-1
      settings: AttributesFormatString=<initial=%<x0>>
  Unit Delay1 : UnitDelay  InitialCondition=1  SampleTime=-1
      settings: AttributesFormatString=<initial=%<x0>>
  Q : Outport
  wires:
  S/1 -> OR/1
  Unit Delay/1 -> Switch/3
  R/1 -> NOT/1
  NOT/1 -> AND/1
  OR/1 -> AND/2
  AND/1 -> Unit Delay/1, Q/1
  Switch/1 -> OR/2
  IV/1 -> Switch/1
  Unit Delay1/1 -> Switch/2
  Constant/1 -> Unit Delay1/1

== system HY_General_Library/Debounce_Blocks/Debounce_Cnt/TurnOnDelayCnt ==
  u : Inport
  Cnt : Inport  Port=2
  Constant1 : Constant  Value=0  OutDataTypeStr=Inherit: Inherit via back propagation
  Constant2 : Constant  OutDataTypeStr=Inherit: Inherit via back propagation
  Constant3 : Constant  Value=0  OutDataTypeStr=Inherit: Inherit via back propagation
  Data Type Duplicate : DataTypeDuplicate  NumInputPorts=4
  Logical Operator : Logic  OutDataTypeStr=boolean
  Logical Operator1 : Logic  OutDataTypeStr=boolean
  Logical Operator2 : Logic  Operator=NOT  OutDataTypeStr=boolean
  RelationalOperator : RelationalOperator  RndMeth=Nearest  InputSameDT=on
  Sum : Sum  SaturateOnIntegerOverflow=on
  Switch1 : Switch  Criteria=u2 ~= 0  SaturateOnIntegerOverflow=on  InputSameDT=on
      settings: AttributesFormatString=%<Criteria>
  Switch4 : Switch  Criteria=u2 ~= 0  SaturateOnIntegerOverflow=on  InputSameDT=on
      settings: AttributesFormatString=%<Criteria>
  Unit Delay : UnitDelay  SampleTime=-1
      settings: AttributesFormatString=Init: %<X0>
  Unit Delay1 : UnitDelay  SampleTime=-1
      settings: AttributesFormatString=Init: %<X0>
  y : Outport
  wires:
  u/1 -> Logical Operator1/2, [u]
  RelationalOperator/1 -> Unit Delay1/1, Logical Operator/1
  Logical Operator/1 -> y/1
  Sum/1 -> RelationalOperator/1, Unit Delay/1
  Cnt/1 -> Data Type Duplicate/1, RelationalOperator/2
  Unit Delay1/1 -> Logical Operator2/1
  Logical Operator1/1 -> Switch4/2
  Logical Operator2/1 -> Logical Operator1/1
  Constant1/1 -> Data Type Duplicate/4, Switch4/3
  Constant2/1 -> Data Type Duplicate/3, Switch4/1
  Switch4/1 -> Sum/2
  Unit Delay/1 -> Switch1/1
  [u] -> Switch1/2
  Constant3/1 -> Data Type Duplicate/2, Switch1/3
  Switch1/1 -> Sum/1
  [u] -> Logical Operator/2

== system HY_General_Library/Debounce_Blocks/Debounce_Cnt/TurnOnDelayCnt1 ==
  u : Inport
  Cnt : Inport  Port=2
  Constant1 : Constant  Value=0  OutDataTypeStr=Inherit: Inherit via back propagation
  Constant2 : Constant  OutDataTypeStr=Inherit: Inherit via back propagation
  Constant3 : Constant  Value=0  OutDataTypeStr=Inherit: Inherit via back propagation
  Data Type Duplicate : DataTypeDuplicate  NumInputPorts=4
  Logical Operator : Logic  OutDataTypeStr=boolean
  Logical Operator1 : Logic  OutDataTypeStr=boolean
  Logical Operator2 : Logic  Operator=NOT  OutDataTypeStr=boolean
  RelationalOperator : RelationalOperator  RndMeth=Nearest  InputSameDT=on
  Sum : Sum  SaturateOnIntegerOverflow=on
  Switch1 : Switch  Criteria=u2 ~= 0  SaturateOnIntegerOverflow=on  InputSameDT=on
      settings: AttributesFormatString=%<Criteria>
  Switch4 : Switch  Criteria=u2 ~= 0  SaturateOnIntegerOverflow=on  InputSameDT=on
      settings: AttributesFormatString=%<Criteria>
  Unit Delay : UnitDelay  SampleTime=-1
      settings: AttributesFormatString=Init: %<X0>
  Unit Delay1 : UnitDelay  SampleTime=-1
      settings: AttributesFormatString=Init: %<X0>
  y : Outport
  wires:
  [u] -> Logical Operator/2
  Switch1/1 -> Sum/1
  Constant3/1 -> Switch1/3, Data Type Duplicate/2
  [u] -> Switch1/2
  Unit Delay/1 -> Switch1/1
  Switch4/1 -> Sum/2
  Constant2/1 -> Switch4/1, Data Type Duplicate/3
  Constant1/1 -> Switch4/3, Data Type Duplicate/4
  Logical Operator2/1 -> Logical Operator1/1
  Logical Operator1/1 -> Switch4/2
  Unit Delay1/1 -> Logical Operator2/1
  Cnt/1 -> RelationalOperator/2, Data Type Duplicate/1
  Sum/1 -> Unit Delay/1, RelationalOperator/1
  Logical Operator/1 -> y/1
  RelationalOperator/1 -> Logical Operator/1, Unit Delay1/1
  u/1 -> [u], Logical Operator1/2

== system HY_General_Library/Debounce_Blocks/Debounce_OBD_FCN/Debounce_OBD ==
  bErr : Inport
  bRst : Inport  Port=2
  FailThd : Inport  Port=3
  RecThd : Inport  Port=4
  IncrFail : Inport  Port=5
  DecrRec : Inport  Port=6
  Enable : EnablePort
  Constant1 : Constant  Value=0  OutDataTypeStr=Inherit: Inherit via back propagation
  Relay : Subsystem
  Sum1 : Sum  OutDataTypeStr=int16  SaturateOnIntegerOverflow=on
  Sum2 : Sum  OutDataTypeStr=int16  SaturateOnIntegerOverflow=on
  Switch1 : Switch  Criteria=u2 ~= 0  OutDataTypeStr=int16  SaturateOnIntegerOverflow=on
  Switch2 : Switch  Criteria=u2 ~= 0  SaturateOnIntegerOverflow=on
  Switch4 : Switch  Criteria=u2 ~= 0  SaturateOnIntegerOverflow=on
  Unit Delay : UnitDelay  SampleTime=-1
      settings: AttributesFormatString=<initial=%<X0>>
  counterRst : Subsystem
  bOutRanged : Outport  InitialOutput=0
  bFailed : Outport  Port=2  InitialOutput=0
  wires:
  IncrFail/1 -> Sum1/1
  DecrRec/1 -> Sum2/1
  Switch2/1 -> Unit Delay/1
  Relay/2(outRanged) -> Switch2/2, bOutRanged/1
  Sum2/1 -> Switch1/3
  Sum1/1 -> Switch1/1
  RecThd/1 -> Relay/2(RecThd)
  FailThd/1 -> Relay/1(FailThd)
  bRst/1 -> Relay/3(Rst), [bRst]
  Relay/1(bFailed) -> bFailed/1
  Unit Delay/1 -> counterRst/2(z_1)
  bErr/1 -> Switch1/2, counterRst/1(bErr)
  Constant1/1 -> Switch4/1
  counterRst/1(O) -> Switch4/3
  Switch4/1 -> Switch2/1, Sum2/2, Sum1/2
  [bRst] -> Switch4/2
  Switch1/1 -> Relay/4(errCtr), Switch2/3

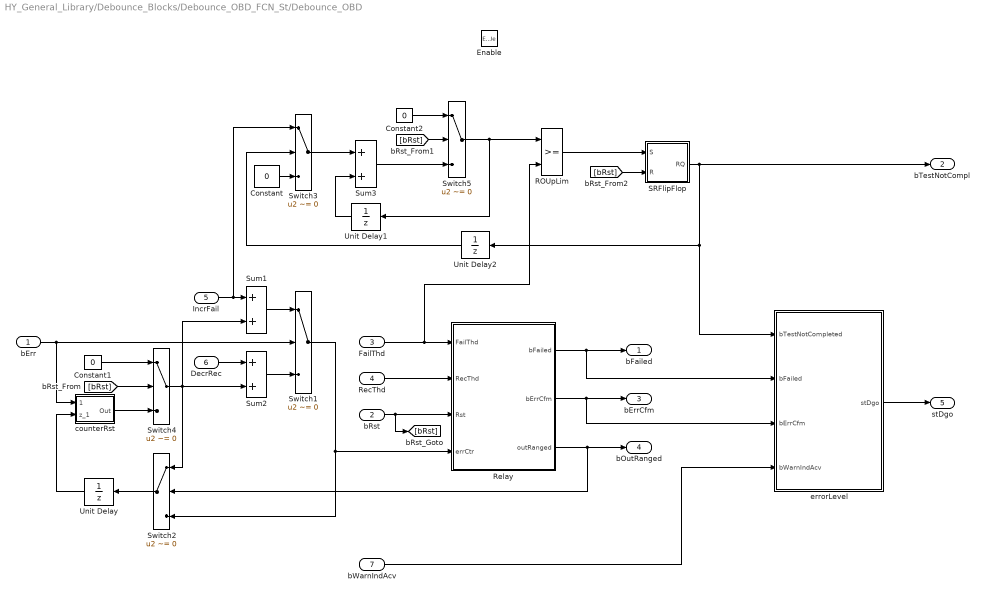
== system HY_General_Library/Debounce_Blocks/Debounce_OBD_FCN_St/Debounce_OBD ==
  bErr : Inport
  bRst : Inport  Port=2
  FailThd : Inport  Port=3
  RecThd : Inport  Port=4
  IncrFail : Inport  Port=5
  DecrRec : Inport  Port=6
  bWarnIndAcv : Inport  Port=7
  Enable : EnablePort
  Constant : Constant  Value=0  OutDataTypeStr=Inherit: Inherit via back propagation
  Constant1 : Constant  Value=0  OutDataTypeStr=Inherit: Inherit via back propagation
  Constant2 : Constant  Value=0  OutDataTypeStr=Inherit: Inherit via back propagation
  ROUpLim : RelationalOperator  OutDataTypeStr=boolean  RndMeth=Nearest
  Relay : Subsystem
  SRFlipFlop : Subsystem
  Sum1 : Sum  OutDataTypeStr=int16  SaturateOnIntegerOverflow=on
  Sum2 : Sum  OutDataTypeStr=int16  SaturateOnIntegerOverflow=on
  Sum3 : Sum  OutDataTypeStr=int16  SaturateOnIntegerOverflow=on
  Switch1 : Switch  Criteria=u2 ~= 0  OutDataTypeStr=int16  SaturateOnIntegerOverflow=on
  Switch2 : Switch  Criteria=u2 ~= 0  SaturateOnIntegerOverflow=on
  Switch3 : Switch  Criteria=u2 ~= 0  SaturateOnIntegerOverflow=on
  Switch4 : Switch  Criteria=u2 ~= 0  SaturateOnIntegerOverflow=on
  Switch5 : Switch  Criteria=u2 ~= 0  OutDataTypeStr=int16  SaturateOnIntegerOverflow=on
  Unit Delay : UnitDelay  SampleTime=-1
      settings: AttributesFormatString=Init: %<X0>
  Unit Delay1 : UnitDelay  SampleTime=-1
      settings: AttributesFormatString=Init: %<X0>
  Unit Delay2 : UnitDelay  SampleTime=-1
      settings: AttributesFormatString=Init: %<X0>
  counterRst : Subsystem
  errorLevel : Subsystem
  bFailed : Outport  InitialOutput=0
  bTestNotCompl : Outport  Port=2  InitialOutput=1
  bErrCfm : Outport  Port=3  InitialOutput=0
  bOutRanged : Outport  Port=4  InitialOutput=0
  stDgo : Outport  Port=5  InitialOutput=0
  wires:
  [bRst] -> SRFlipFlop/2(R)
  Switch1/1 -> Switch2/3, Relay/4(errCtr)
  [bRst] -> Switch5/2
  Constant2/1 -> Switch5/1
  Switch5/1 -> ROUpLim/1, Unit Delay1/1
  Sum3/1 -> Switch5/3
  [bRst] -> Switch4/2
  Switch4/1 -> Sum1/2, Sum2/2, Switch2/1
  counterRst/1(Out) -> Switch4/3
  Constant1/1 -> Switch4/1
  bErr/1 -> counterRst/1(bErr), Switch1/2
  Unit Delay/1 -> counterRst/2(z_1)
  Relay/1(bFailed) -> bFailed/1, errorLevel/2(bFailed)
  bRst/1 -> [bRst], Relay/3(Rst)
  Relay/2(bErrCfm) -> bErrCfm/1, errorLevel/3(bErrCfm)
  FailThd/1 -> ROUpLim/2, Relay/1(FailThd)
  RecThd/1 -> Relay/2(RecThd)
  Sum1/1 -> Switch1/1
  Sum2/1 -> Switch1/3
  Relay/3(outRanged) -> Switch2/2, bOutRanged/1
  Switch2/1 -> Unit Delay/1
  DecrRec/1 -> Sum2/1
  IncrFail/1 -> Sum1/1, Switch3/1
  Unit Delay1/1 -> Sum3/2
  ROUpLim/1 -> SRFlipFlop/1(S)
  SRFlipFlop/1(RQ) -> bTestNotCompl/1, errorLevel/1(bTestNotCompleted), Unit Delay2/1
  Switch3/1 -> Sum3/1
  Constant/1 -> Switch3/3
  Unit Delay2/1 -> Switch3/2
  bWarnIndAcv/1 -> errorLevel/4(bWarnIndAcv)
  errorLevel/1(stDgo) -> stDgo/1

== system HY_General_Library/Filter_Blocks/Average_LPF/Limit ==
  MX : Inport
  u : Inport  Port=2
  MN : Inport  Port=3
  MinMax10 : MinMax  Function=max  Inputs=2
  MinMax5 : MinMax  Inputs=2
  y : Outport
  wires:
  MinMax5/1 -> y/1
  MinMax10/1 -> MinMax5/1
  u/1 -> MinMax10/1
  MN/1 -> MinMax10/2
  MX/1 -> MinMax5/2

== system HY_General_Library/Filter_Blocks/DT1/IniCdn1 ==
  In : Inport
  Ini : Inport  Port=2
  Constant3 : Constant  OutDataTypeStr=boolean  SampleTime=-1
  Switch : Switch  Criteria=u2 ~= 0  SaturateOnIntegerOverflow=on  InputSameDT=on
      settings: AttributesFormatString=threshold=%<threshold>\nCriteria : %<Criteria>
  UnitDelay : UnitDelay  SampleTime=-1
      settings: AttributesFormatString=dT = %<SampleTime>\nIni=%<X0>
  Out : Outport
  wires:
  Switch/1 -> Out/1
  Constant3/1 -> UnitDelay/1
  UnitDelay/1 -> Switch/2
  Ini/1 -> Switch/3
  In/1 -> Switch/1

== system HY_General_Library/Filter_Blocks/DT1/UnitDly_ExtIni2 ==
  u : Inport
  RV : Inport  Port=2
  Constant3 : Constant  OutDataTypeStr=boolean  SampleTime=-1
  Switch : Switch  Criteria=u2 ~= 0  SaturateOnIntegerOverflow=on  InputSameDT=on
      settings: AttributesFormatString=|
      | %<Criteria>
      | threshold=%<threshold>
  UnitDelay : UnitDelay  SampleTime=-1  StateName=UnitDelay
      settings: AttributesFormatString=Init=%<X0>
  UnitDelay1 : UnitDelay  SampleTime=-1  StateName=UnitDelay
      settings: AttributesFormatString=Init=%<X0>
  y : Outport
  wires:
  RV/1 -> Switch/3
  Switch/1 -> y/1
  u/1 -> UnitDelay/1
  Constant3/1 -> UnitDelay1/1
  UnitDelay1/1 -> Switch/2
  UnitDelay/1 -> Switch/1

== system HY_General_Library/Filter_Blocks/DT1/UnitDly_ExtIni3 ==
  In : Inport
  Ini : Inport  Port=2
  Constant3 : Constant  OutDataTypeStr=boolean  SampleTime=-1
  Switch : Switch  Criteria=u2 ~= 0  SaturateOnIntegerOverflow=on  InputSameDT=on
      settings: AttributesFormatString=threshold=%<threshold>\nCriteria : %<Criteria>
  UnitDelay : UnitDelay  SampleTime=-1  StateName=UnitDelay
      settings: AttributesFormatString=|
      | UnitDelay
      | dT = %<SampleTime>\nIni=%<X0>
  UnitDelay1 : UnitDelay  SampleTime=-1  StateName=UnitDelay
      settings: AttributesFormatString=|
      | UnitDelay
      | dT = %<SampleTime>\nIni=%<X0>
  Out : Outport
  wires:
  UnitDelay/1 -> Switch/1
  UnitDelay1/1 -> Switch/2
  Constant3/1 -> UnitDelay1/1
  In/1 -> UnitDelay/1
  Switch/1 -> Out/1
  Ini/1 -> Switch/3

== system HY_General_Library/Filter_Blocks/LPF1_K/LIMIT ==
  Max : Inport
  u : Inport  Port=2
  Min : Inport  Port=3
  Data Type Propagation : simulink/Signal Attributes/Data Type Propagation  PropDataType=fixdt(1, 16)  IfRefDouble=double  IfRefSingle=single  IsSigned=IsSigned1  NumBitsBase=NumBits1  NumBitsMult=1  NumBitsAdd=0  NumBitsAllowFinal=1:128  PropScaling=2^-10  ValuesUsedBestPrec=[5 -7]  SlopeBase=min([Slope1 Slope2])  SlopeMult=1  SlopeAdd=0  BiasBase=Bias1  BiasMult=1  BiasAdd=0
      settings: SourceProductName=Simulink  SourceProductBaseCode=SL
  Data Type Propagation1 : simulink/Signal Attributes/Data Type Propagation  PropDataType=fixdt(1, 16)  IfRefDouble=double  IfRefSingle=single  IsSigned=IsSigned1  NumBitsBase=NumBits1  NumBitsMult=1  NumBitsAdd=0  NumBitsAllowFinal=1:128  PropScaling=2^-10  ValuesUsedBestPrec=[5 -7]  SlopeBase=min([Slope1 Slope2])  SlopeMult=1  SlopeAdd=0  BiasBase=Bias1  BiasMult=1  BiasAdd=0
      settings: SourceProductName=Simulink  SourceProductBaseCode=SL
  MinMax : MinMax  Inputs=2  SaturateOnIntegerOverflow=on  InputSameDT=on
  MinMax1 : MinMax  Function=max  Inputs=2  OutDataTypeStr=Inherit: Inherit via back propagation  SaturateOnIntegerOverflow=on
  y : Outport  InitialOutput=0
  wires:
  Max/1 -> MinMax/1
  u/1 -> MinMax1/1, Data Type Propagation1/1, Data Type Propagation1/2, Data Type Propagation/1, Data Type Propagation/2
  Min/1 -> MinMax1/2
  MinMax1/1 -> Data Type Propagation/3, MinMax/2
  MinMax/1 -> Data Type Propagation1/3, y/1

== system HY_General_Library/PID_Blocks/PositionPID/Subsystem1 ==
  Reset : Inport
  PreSat : Inport  Port=2
  UpperSatLimd : Inport  Port=3
  Err : Inport  Port=4
  CtrlIntgVal : Inport  Port=5
  ResetVal : Inport  Port=6
  LowerSatLimd : Inport  Port=7
  Add1 : Sum
  Multiport Switch : MultiPortSwitch  DataPortOrder=Zero-based contiguous  Inputs=2  zeroidx=on
  Subsystem : Subsystem
  Unit Delay : UnitDelay  SampleTime=-1
  Out : Outport
  wires:
  PreSat/1 -> Subsystem/2(PreSat)
  UpperSatLimd/1 -> Subsystem/3(UpperSatLimd)
  Err/1 -> Subsystem/1(Err)
  Reset/1 -> Multiport Switch/1
  Add1/1 -> Multiport Switch/2
  ResetVal/1 -> Multiport Switch/3
  Multiport Switch/1 -> Unit Delay/1
  CtrlIntgVal/1 -> Subsystem/5(CtrlIntgVal)
  Subsystem/1(Out) -> Add1/1
  Unit Delay/1 -> Add1/2, Out/1
  LowerSatLimd/1 -> Subsystem/4(LowerSatLimd)

== system HY_General_Library/Debounce_Blocks/Debounce_OBD_FCN/Debounce_OBD/Relay ==
  note: FailCtr <= errCtr <= RecoverCtr
  FailThd : Inport
  RecThd : Inport  Port=2
  Rst : Inport  Port=3
  errCtr : Inport  Port=4
  LORelay : Logic  Operator=OR  AllPortsSameDT=off  OutDataTypeStr=boolean
  LORelay1 : Logic  Operator=OR  AllPortsSameDT=off  OutDataTypeStr=boolean
  ROLoLim : RelationalOperator  Operator=<=  OutDataTypeStr=boolean  RndMeth=Nearest
  ROUpLim : RelationalOperator  Operator=<=  OutDataTypeStr=boolean  RndMeth=Nearest
  SRFlipFlop : Subsystem
  bFailed : Outport
  outRanged : Outport  Port=2
  wires:
  Rst/1 -> LORelay1/2
  RecThd/1 -> ROLoLim/2
  SRFlipFlop/1(Q) -> bFailed/1
  LORelay/1 -> outRanged/1  "outRanged"
  errCtr/1 -> ROLoLim/1, ROUpLim/2
  ROLoLim/1 -> LORelay/2, LORelay1/1
  ROUpLim/1 -> SRFlipFlop/1(S), LORelay/1
  FailThd/1 -> ROUpLim/1
  LORelay1/1 -> SRFlipFlop/2(R)

== system HY_General_Library/Debounce_Blocks/Debounce_OBD_FCN/Debounce_OBD/counterRst ==
  note: test run failure always causes fault detection counter to increment above 0
      | (so as not to double the fail detection time following a test complete with pass)
  note: only if the FaultDetectionCounter less than 0
  note: rising edge detection
  bErr : Inport
  z_1 : Inport  Port=2
  ConstOne1 : Constant  Description=TOPexpert TAT block library for modelling of ECU functions - (c) by FEV - all rights reserved. Confidential - no passing on third parties, Calibration Methods (TEM), 2003-2006, schoenfelder  InitFcn=try;p = get_param(gcb,'Ports'); p = p(1);posblk = get_param(gcb,'Position');set_param(gcb,'Position',[posblk(1) posblk(2) posblk(1)+25 posblk(2)+15]);end;  Value=0  OutDataTypeStr=int16
      settings: PreSaveFcn=try;p = get_param(gcb,'Ports'); p = p(1);posblk = get_param(gcb,'Position');set_param(gcb,'Position',[posblk(1) posblk(2) posblk(1)+25 posblk(2)+15]);end;
  ConstOne10 : Constant  Description=TOPexpert TAT block library for modelling of ECU functions - (c) by FEV - all rights reserved. Confidential - no passing on third parties, Calibration Methods (TEM), 2003-2006, schoenfelder  InitFcn=try;p = get_param(gcb,'Ports'); p = p(1);posblk = get_param(gcb,'Position');set_param(gcb,'Position',[posblk(1) posblk(2) posblk(1)+25 posblk(2)+15]);end;  Value=0  OutDataTypeStr=int16
      settings: PreSaveFcn=try;p = get_param(gcb,'Ports'); p = p(1);posblk = get_param(gcb,'Position');set_param(gcb,'Position',[posblk(1) posblk(2) posblk(1)+25 posblk(2)+15]);end;
  Logical Operator : Logic  AllPortsSameDT=off  OutDataTypeStr=boolean
  Relational Operator : RelationalOperator  Operator=<  OutDataTypeStr=boolean  RndMeth=Nearest
  Relational Operator1 : RelationalOperator  Operator=>  OutDataTypeStr=boolean  RndMeth=Nearest  InputSameDT=on
  SwCtrResetDurFail : Switch  Criteria=u2 ~= 0  SaturateOnIntegerOverflow=on
  Unit Delay1 : UnitDelay  SampleTime=-1
      settings: AttributesFormatString=<initial=%<X0>>
  O : Outport
  wires:
  SwCtrResetDurFail/1 -> O/1
  bErr/1 -> Unit Delay1/1, Relational Operator1/1
  Logical Operator/1 -> SwCtrResetDurFail/2
  Relational Operator/1 -> Logical Operator/2
  ConstOne10/1 -> Relational Operator/2
  Relational Operator1/1 -> Logical Operator/1
  Unit Delay1/1 -> Relational Operator1/2
  ConstOne1/1 -> SwCtrResetDurFail/1
  z_1/1 -> Relational Operator/1, SwCtrResetDurFail/3

== system HY_General_Library/Debounce_Blocks/Debounce_OBD_FCN_St/Debounce_OBD/Relay ==
  note: FailCtr <= errCtr <= RecoverCtr
  FailThd : Inport
  RecThd : Inport  Port=2
  Rst : Inport  Port=3
  errCtr : Inport  Port=4
  LORelay : Logic  Operator=OR  AllPortsSameDT=off  OutDataTypeStr=boolean
  LORelay1 : Logic  Operator=OR  AllPortsSameDT=off  OutDataTypeStr=boolean
  ROLoLim : RelationalOperator  Operator=<=  OutDataTypeStr=boolean  RndMeth=Nearest
  ROUpLim : RelationalOperator  Operator=<=  OutDataTypeStr=boolean  RndMeth=Nearest
  SRFlipFlop : Subsystem
  SRFlipFlop1 : Subsystem
  bFailed : Outport
  bErrCfm : Outport  Port=2
  outRanged : Outport  Port=3
  wires:
  LORelay1/1 -> SRFlipFlop/2(R)
  FailThd/1 -> ROUpLim/1
  ROUpLim/1 -> SRFlipFlop/1(S), LORelay/1
  ROLoLim/1 -> LORelay1/1, LORelay/2
  errCtr/1 -> ROUpLim/2, ROLoLim/1
  LORelay/1 -> outRanged/1
  SRFlipFlop/1(Q) -> SRFlipFlop1/1(S), bFailed/1
  SRFlipFlop1/1(Q) -> bErrCfm/1
  RecThd/1 -> ROLoLim/2
  Rst/1 -> SRFlipFlop1/2(R), LORelay1/2

== system HY_General_Library/Debounce_Blocks/Debounce_OBD_FCN_St/Debounce_OBD/SRFlipFlop ==
  note: Vectorized SR Flip Flop
  S : Inport
  R : Inport  Port=2
  SRNOR : Logic  Operator=NOR  AllPortsSameDT=off  OutDataTypeStr=boolean
  SRNOR1 : Logic  Operator=NOR  AllPortsSameDT=off  OutDataTypeStr=boolean
  Unit Delay1 : UnitDelay  InitialCondition=1  SampleTime=-1
      settings: AttributesFormatString=<initial=%<X0>>
  RQ : Outport
  wires:
  Unit Delay1/1 -> SRNOR1/2
  SRNOR/1 -> Unit Delay1/1, RQ/1
  S/1 -> SRNOR/1
  SRNOR1/1 -> SRNOR/2
  R/1 -> SRNOR1/1
